simulink model "MotorControlLibNEW"  (R2020b)
settings: Solver=FixedStepDiscrete  StartTime=0.0  StopTime=100  FixedStep=Ts  RelTol=1e-3
values from neighbouring files (symbols this model uses):
  Jm = 0.0000008    (= 8e-07)    [MotorControlLibData.m]    (also in local_pmsm_torque_control_data.m)
  Ld = 1.93E-5    [MotorControl.sldd]    (also in MotorControlLibData.m = 1.93e-05; local_pmsm_torque_control_data.m = 1.93e-05)
  p = 4.0    [MotorControl.sldd]    (also in MotorControlLibData.m = 4; local_pmsm_torque_control_data.m = 4)
  psim = 0.00375    [MotorControl.sldd]    (also in MotorControlLibData.m = 0.00375)
  Rs = 0.022    [MotorControl.sldd]    (also in MotorControlLibData.m = 0.022; local_pmsm_torque_control_data.m = 0.022)
  Ts = 5.0E-5    [MotorControl.sldd]    (also in MotorControlLibData.m = 0.00025; local_pmsm_torque_control_data.m = 5e-06)
  Vnom = 12.0    [MotorControl.sldd]    (also in MotorControlLibData.m = 12; local_pmsm_torque_control_data.m = 12)
undefined symbols (not defined in the file or in its folder): DiscIntNeverNeededParam, Down, Up
libraries: mcbcontrolslib x6, pid_lib x4, eePwmGenerator x3, simulink x2, autolibpmsmexterior x1, eeDqVoltageLimiter x1
settings Model: DataDictionary=MotorControl.sldd  NumberOfSteps=36  Creator=unix  LastModifiedBy=unix
settings SolverCC: AutoInsertRateTranBlk=on

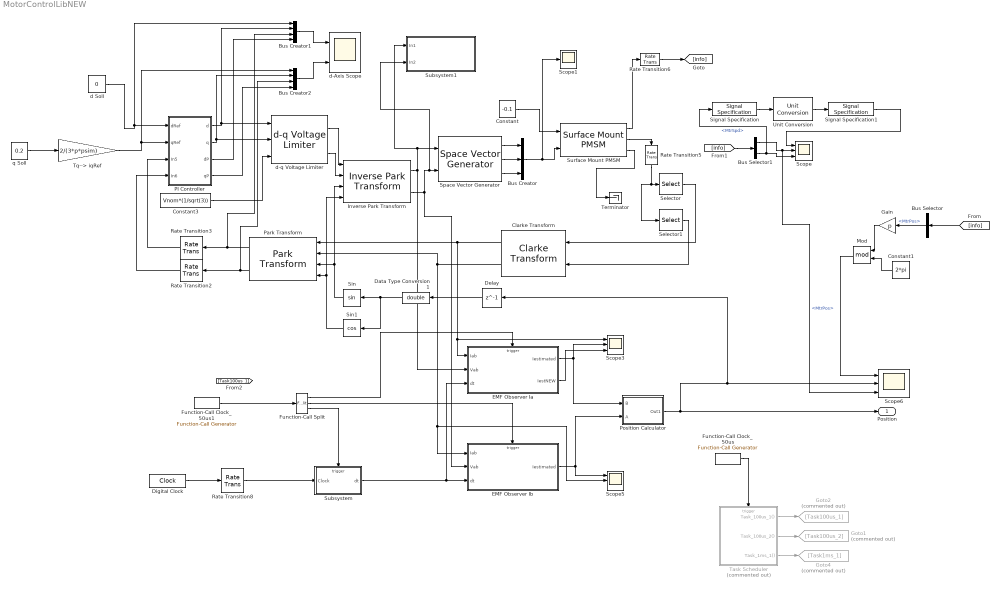
== system MotorControlLibNEW ==
  Bus Creator : BusCreator  Inputs=3
  Bus Creator1 : BusCreator  Inputs=4
  Bus Creator2 : BusCreator  Inputs=4
  Bus Selector : BusSelector  OutputSignals=MtrPos
  Bus Selector1 : BusSelector  OutputSignals=MtrPos,MtrSpd
  Clarke Transform : mcbcontrolslib/Clarke Transform  VariantControl=Variant2
  Constant : Constant  Value=-0.1
  Constant1 : Constant  Value=2*pi
  Constant3 : Constant  Value=Vnom*(1/sqrt(3))
  Data Type Conversion1 : DataTypeConversion  OutDataTypeStr=double
  Delay : Delay  DelayLength=1
  Digital Clock : DigitalClock  SampleTime=Ts
  EMF Observer Ia : Subsystem  mask{Rs=Rs/2, Ld=1/(Ld/2), P=0.255, I=1600}
      mask prompts: Rs "Resistance"; Ld "Inductance"; P "Simulink:masks:ProportionalP_MP"; I "Simulink:masks:IntegralI_MP"
      mask TypeOptions Rs: Resistance/Gain
      mask TypeOptions Ld: Inductance/Gain
      mask TypeOptions P: PID Controller/P
      mask TypeOptions I: PID Controller/I
      mask DialogControl Container6 Prompt: PI Controller
      mask DialogControl P Prompt: Proportional (P):
      mask DialogControl I Prompt: Integral (I):
  EMF Observer Ib : Subsystem  mask{Rs=Rs/2, Ld=1/(Ld/2), P=0.255, I=1600}
      mask prompts: Rs "Resistance"; Ld "Inductance"; P "Simulink:masks:ProportionalP_MP"; I "Simulink:masks:IntegralI_MP"
      mask TypeOptions Rs: Resistance/Gain
      mask TypeOptions Ld: Inductance/Gain
      mask TypeOptions P: PID Controller/P
      mask TypeOptions I: PID Controller/I
      mask DialogControl Container6 Prompt: PI Controller
      mask DialogControl P Prompt: Proportional (P):
      mask DialogControl I Prompt: Integral (I):
  Function-Call Clock_50us : simulink/Ports & Subsystems/Function-Call Generator  sample_time=5e-5  numberOfIterations=1  DisallowWideOutput=off
  Function-Call Clock_50us1 : simulink/Ports & Subsystems/Function-Call Generator  sample_time=Ts  numberOfIterations=1  DisallowWideOutput=off
  Function-Call Split : FunctionCallSplit  IconShape=distinctive  NumOutputPorts=3  OutputPortLayout=default
  Gain : Gain  Gain=p
  Goto1 : Goto  Commented=on  GotoTag=Task100us_2
  Goto2 : Goto  Commented=on  GotoTag=Task100us_1
  Goto4 : Goto  Commented=on  GotoTag=Task1ms_1
  Inverse Park Transform : mcbcontrolslib/Inverse Park Transform  AxisAlignment=D-axis
  Mod : Math  Operator=mod  SaturateOnIntegerOverflow=on
  PI Controller : Subsystem
  Park Transform : mcbcontrolslib/Park Transform  AxisAlignment=D-axis
      settings: SourceProductBaseCode=MT
  Position Calculator : Subsystem
  Rate Transition{2..3,5..6,8} (5 alike) : RateTransition
  Scope{,3,5..6} (4 alike) : Scope  NumInputPorts=3
  Scope1 : Scope
  Selector : Selector  InputPortWidth=3  IndexOptions=Index vector (dialog)  Indices=1  OutputSizes=1
  Selector1 : Selector  InputPortWidth=3  IndexOptions=Index vector (dialog)  Indices=2  OutputSizes=1
  Signal Specification : SignalSpecification  Unit=rad/s
  Signal Specification1 : SignalSpecification  Unit=rpm
  Sin : Trigonometry
  Sin1 : Trigonometry  Operator=cos
  Space Vector Generator : mcbcontrolslib/Space Vector Generator
      settings: SourceProductBaseCode=MT
  Subsystem : Subsystem
  Subsystem1 : Subsystem
  Surface Mount PMSM : autolibpmsmexterior/Surface Mount PMSM  port_config=Torque  sim_type=Discrete  Ts=Ts  P=p  Rs=Rs/2  Ldq_=Ld/2  KConstText=Back-emf constant (Ke):  lambda_pm=0.2205  Ke=cBackEMF_VKPRM  Kt=1.323  mechanical=[Jm, 4.924e-4, 0]  idq0=[0 0]  theta_init=0  omega_init=0  KConst=0.2205  lambda_pm_calc=0.0021651  RefBlkName='autolibpmsmexterior/Surface Mount PMSM'  aMode=5  Ldq="[0.0017      0.0017]"
      settings: SourceProductBaseCode=PW,MT,UV,VE,VP
  Task Scheduler : Stateflow chart  Commented=on  TreatAsAtomicUnit=on
  Terminator : Terminator
  Tq--> iqRef : Gain  Gain=2/(3*p*psim)
  Unit Conversion : UnitConversion
  d Soll : Constant  Value=0
  d-Axis Scope : Scope  NumInputPorts=2
  d-q Voltage Limiter : eeDqVoltageLimiter/d-q Voltage Limiter  AxisPrio=D-axis  Ts=-1
      settings: SourceProductBaseCode=PS
  q Soll : Constant  Value=0.2
  Position : Outport
  wires:
  Constant/1 -> Surface Mount PMSM/1
  Selector1/1 -> Clarke Transform/2
  Selector/1 -> Clarke Transform/1
  Clarke Transform/1 -> Scope3/1, EMF Observer Ia/1(Iab), Park Transform/1
  Clarke Transform/2 -> Park Transform/2, EMF Observer Ib/1(Iab), Scope5/2
  [info] -> Bus Selector/1
  Surface Mount PMSM/1 -> Rate Transition6/1
  Bus Selector/1 -> Gain/1  "<MtrPos>"
  Sin/1 -> Inverse Park Transform/3, Park Transform/3
  Sin1/1 -> Park Transform/4, Inverse Park Transform/4
  Inverse Park Transform/1 -> Subsystem1/1(In1), Space Vector Generator/1, EMF Observer Ia/2(Vab)
  Space Vector Generator/2 -> Bus Creator/2
  Space Vector Generator/3 -> Bus Creator/3
  Bus Selector1/2 -> Signal Specification/1, Scope/3  "<MtrSpd>"
  [info] -> Bus Selector1/1
  Bus Selector1/1 -> Scope6/3, Scope/2  "<MtrPos>"
  Surface Mount PMSM/3 -> Terminator/1
  d-q Voltage Limiter/1 -> Inverse Park Transform/1
  d-q Voltage Limiter/2 -> Inverse Park Transform/2
  Constant3/1 -> d-q Voltage Limiter/3
  Signal Specification1/1 -> Scope/1
  Signal Specification/1 -> Unit Conversion/1
  Unit Conversion/1 -> Signal Specification1/1
  Task Scheduler/1(Task_100us_1()) -> Goto2/1
  Function-Call Clock_50us/1 -> Task Scheduler/Trigger
  Task Scheduler/3(Task_1ms_1()) -> Goto4/1
  Task Scheduler/2(Task_100us_2()) -> Goto1/1
  Inverse Park Transform/2 -> Subsystem1/2(In2), Space Vector Generator/2, EMF Observer Ib/2(Vab)
  Function-Call Split/1 -> EMF Observer Ia/Trigger
  Function-Call Split/2 -> EMF Observer Ib/Trigger
  EMF Observer Ia/1(Iestimated) -> Position Calculator/1(B), Scope3/2
  EMF Observer Ib/1(Iestimated) -> Scope5/1, Position Calculator/2(A)
  Surface Mount PMSM/2 -> Rate Transition5/1
  Data Type Conversion1/1 -> Sin/1, Sin1/1
  Delay/1 -> Data Type Conversion1/1
  Digital Clock/1 -> Rate Transition8/1
  Position Calculator/1(Out1) -> Position/1, Delay/1, Scope6/2
  Subsystem/1(dt) -> EMF Observer Ib/3(dt), EMF Observer Ia/3(dt)
  d Soll/1 -> Bus Creator1/1, PI Controller/1(dRef)
  Tq--> iqRef/1 -> Bus Creator2/1, PI Controller/2(qRef)
  Park Transform/1 -> Bus Creator1/3, Rate Transition3/1
  Park Transform/2 -> Rate Transition2/1, Bus Creator2/3
  PI Controller/1(d) -> d-q Voltage Limiter/1, Bus Creator1/2
  PI Controller/2(q) -> d-q Voltage Limiter/2, Bus Creator2/2
  Rate Transition2/1 -> PI Controller/4(In6)
  Rate Transition3/1 -> PI Controller/3(In5)
  Rate Transition5/1 -> Selector1/1, Selector/1
  Rate Transition6/1 -> [info]
  Rate Transition8/1 -> Subsystem/1(Clock)
  Function-Call Split/3 -> Subsystem/Trigger
  Bus Creator1/1 -> d-Axis Scope/1
  Bus Creator2/1 -> d-Axis Scope/2
  Constant1/1 -> Mod/2
  Gain/1 -> Mod/1
  Mod/1 -> Scope6/1
  PI Controller/3(dP) -> Bus Creator1/4
  PI Controller/4(qP) -> Bus Creator2/4
  q Soll/1 -> Tq--> iqRef/1
  EMF Observer Ia/2(IestNEW) -> Scope3/3
  Function-Call Clock_50us1/1 -> Function-Call Split/1
  Bus Creator/1 -> Scope1/1, Surface Mount PMSM/2
  Space Vector Generator/1 -> Bus Creator/1

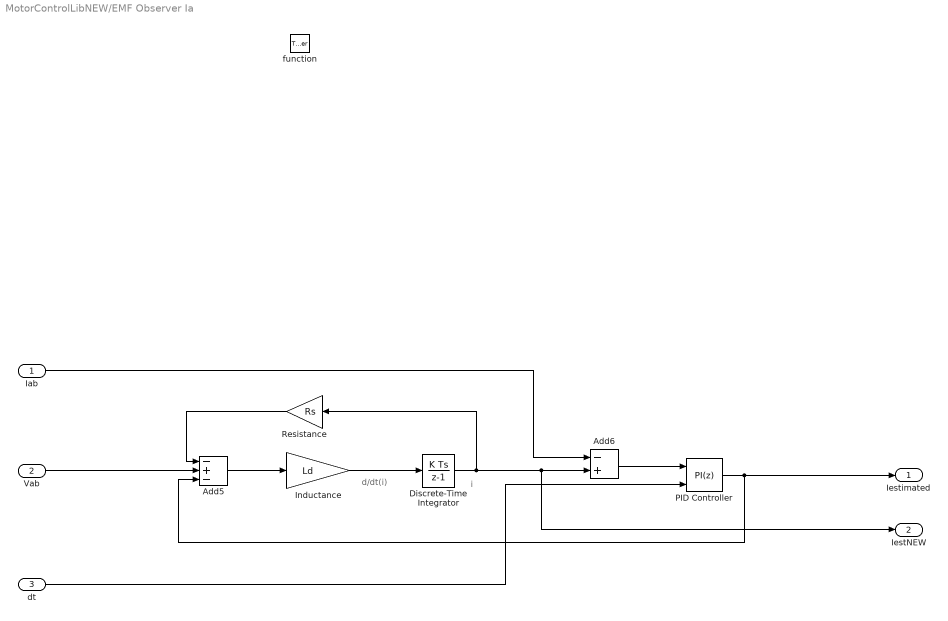
== system MotorControlLibNEW/EMF Observer Ia ==
  note: d/dt(i)
  note: i
  Iab : Inport
  Vab : Inport  Port=2
  dt : Inport  Port=3
  function : TriggerPort  TriggerType=function-call  VariantControl=Variant
  Add5 : Sum  Inputs=-+-
  Add6 : Sum  Inputs=-+
  Discrete-Time Integrator : DiscreteIntegrator  gainval=1  SampleTime=-1  OutDataTypeStr=fixdt(1,32,2^-12,0)  UpperSaturationLimit=18  LowerSaturationLimit=-18  ICPrevOutput=DiscIntNeverNeededParam  ICPrevScaledInput=DiscIntNeverNeededParam
  Inductance : Gain  Gain=Ld
  PID Controller : pid_lib/PID Controller  Controller=PI  Form=Parallel  TimeDomain=Discrete-time  UseExternalTs=on  SampleTime=-1  IntegratorMethod=Forward Euler  FilterMethod=Forward Euler  ControllerParametersSource=internal  P=P  I=I  D=0  UseFilter=on  N=100  TunerSelectOption=Transfer Function Based (PID Tuner App)  InitialConditionSource=internal  InitialConditionForIntegrator=0  InitialConditionForFilter=0  DifferentiatorICPrevScaledInput=0  ExternalReset=none  TrackingMode=off  Kt=1  LimitOutput=off  SatLimitsSource=internal  UpperSaturationLimit=inf  LowerSaturationLimit=-inf  LinearizeAsGain=on  AntiWindupMode=none  Kb=1  POutMin=[]  POutMax=[]  IOutMin=[]  IOutMax=[]  DOutMin=[]  DOutMax=[]  NOutMin=[]  NOutMax=[]  SumOutMin=[]  SumOutMax=[]  SaturationOutMin=[]  SaturationOutMax=[]  PParamMin=[]  PParamMax=[]  IParamMin=[]  IParamMax=[]  DParamMin=[]  DParamMax=[]  NParamMin=[]  NParamMax=[]  KbParamMin=[]  KbParamMax=[]  KtParamMin=[]  KtParamMax=[]  KbOutMin=[]  KbOutMax=[]  KtOutMin=[]  KtOutMax=[]  IntegratorOutMin=[]  IntegratorOutMax=[]  FilterOutMin=[]  FilterOutMax=[]  SumI1OutMin=[]  SumI1OutMax=[]  SumI2OutMin=[]  SumI2OutMax=[]  SumI3OutMin=[]  SumI3OutMax=[]  SumI4OutMin=[]  SumI4OutMax=[]  SumDOutMin=[]  SumDOutMax=[]  DifferentiatorOutMin=[]  DifferentiatorOutMax=[]  FilterDiffOutCoefMin=[]  FilterDiffOutCoefMax=[]  ReciprocalOutMin=[]  ReciprocalOutMax=[]  SumDenOutMin=[]  SumDenOutMax=[]  SumNumOutMin=[]  SumNumOutMax=[]  DivideOutMin=[]  DivideOutMax=[]  UdiffTsProdOutMin=[]  UdiffTsProdOutMax=[]  NTsProdOutMin=[]  NTsProdOutMax=[]  UintegralTsProdOutMin=[]  UintegralTsProdOutMax=[]  UngainTsProdOutMin=[]  UngainTsProdOutMax=[]  IntegratorContinuousStateAttributes=''  IntegratorStateMustResolveToSignalObject=off  IntegratorRTWStateStorageClass=Auto  FilterContinuousStateAttributes=''  FilterStateMustResolveToSignalObject=off  FilterRTWStateStorageClass=Auto  ParallelPVariant=InternalParameters  IdealPVariant=Disabled  IVariant=InternalParameters  DVariant=Disabled  IntegratorVariant=Discrete  SatVariant=Disabled  AWVariant=Passthrough  PCopyVariant=Disabled  TRVariant=Disabled  FdbkBlocksVariant=Forward  IdealPFdbkVariant=Disabled  SatFdbkVariant=Disabled  DerivativeFilterVariant=Disabled  NVariant=Disabled  NCopyVariant=Disabled_SignalSpec  FilterICVariant=Disabled  IntegratorICVariant=InternalICs  ExternalResetVariant=Disabled  TRSumVariant=Passthrough  SumFdbkVariant=Disabled  SumVariant=Sum_PI  TsampFilterVariant=InternalTs  TsampNgainVariant=Passthrough  TsampIntegralVariant=ExternalTs  ExternalSaturationOutDataTypeStr=Inherit: Same as second input
  Resistance : Gain  Gain=Rs
  Iestimated : Outport
  IestNEW : Outport  Port=2
  wires:
  Iab/1 -> Add6/1
  Resistance/1 -> Add5/1
  Add5/1 -> Inductance/1
  Vab/1 -> Add5/2
  Inductance/1 -> Discrete-Time Integrator/1
  Discrete-Time Integrator/1 -> IestNEW/1, Add6/2, Resistance/1
  Add6/1 -> PID Controller/1
  PID Controller/1 -> Add5/3, Iestimated/1
  dt/1 -> PID Controller/2

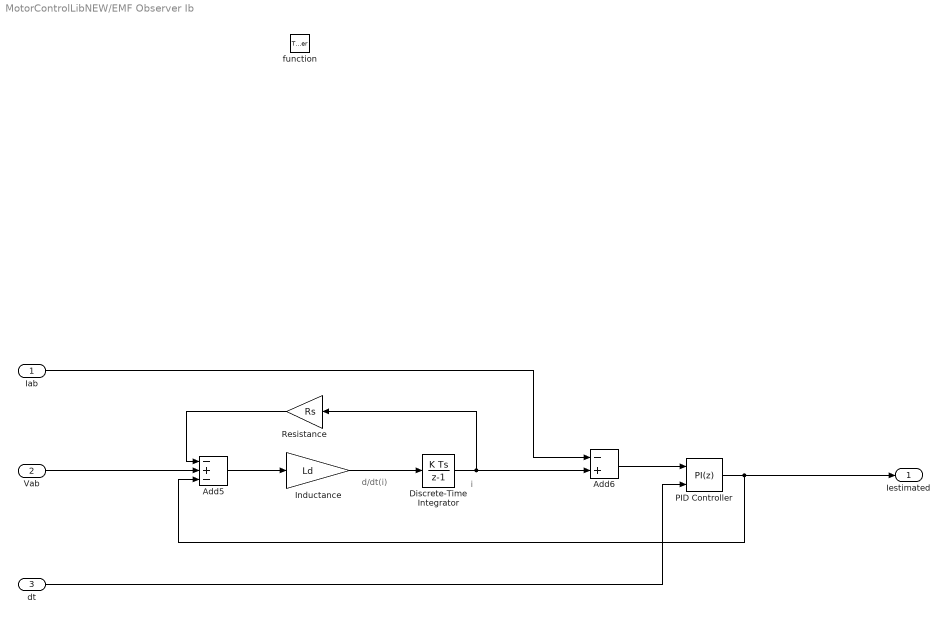
== system MotorControlLibNEW/EMF Observer Ib ==
  note: i
  note: d/dt(i)
  Iab : Inport
  Vab : Inport  Port=2
  dt : Inport  Port=3
  function : TriggerPort  TriggerType=function-call  VariantControl=Variant
  Add5 : Sum  Inputs=-+-
  Add6 : Sum  Inputs=-+
  Discrete-Time Integrator : DiscreteIntegrator  gainval=1  SampleTime=-1  OutDataTypeStr=fixdt(1,32,2^-12,0)  UpperSaturationLimit=18  LowerSaturationLimit=-18  ICPrevOutput=DiscIntNeverNeededParam  ICPrevScaledInput=DiscIntNeverNeededParam
  Inductance : Gain  Gain=Ld
  PID Controller : pid_lib/PID Controller  Controller=PI  Form=Parallel  TimeDomain=Discrete-time  UseExternalTs=on  SampleTime=-1  IntegratorMethod=Forward Euler  FilterMethod=Forward Euler  ControllerParametersSource=internal  P=P  I=I  D=0  UseFilter=on  N=100  TunerSelectOption=Transfer Function Based (PID Tuner App)  InitialConditionSource=internal  InitialConditionForIntegrator=0  InitialConditionForFilter=0  DifferentiatorICPrevScaledInput=0  ExternalReset=none  TrackingMode=off  Kt=1  LimitOutput=off  SatLimitsSource=internal  UpperSaturationLimit=inf  LowerSaturationLimit=-inf  LinearizeAsGain=on  AntiWindupMode=none  Kb=1  POutMin=[]  POutMax=[]  IOutMin=[]  IOutMax=[]  DOutMin=[]  DOutMax=[]  NOutMin=[]  NOutMax=[]  SumOutMin=[]  SumOutMax=[]  SaturationOutMin=[]  SaturationOutMax=[]  PParamMin=[]  PParamMax=[]  IParamMin=[]  IParamMax=[]  DParamMin=[]  DParamMax=[]  NParamMin=[]  NParamMax=[]  KbParamMin=[]  KbParamMax=[]  KtParamMin=[]  KtParamMax=[]  KbOutMin=[]  KbOutMax=[]  KtOutMin=[]  KtOutMax=[]  IntegratorOutMin=[]  IntegratorOutMax=[]  FilterOutMin=[]  FilterOutMax=[]  SumI1OutMin=[]  SumI1OutMax=[]  SumI2OutMin=[]  SumI2OutMax=[]  SumI3OutMin=[]  SumI3OutMax=[]  SumI4OutMin=[]  SumI4OutMax=[]  SumDOutMin=[]  SumDOutMax=[]  DifferentiatorOutMin=[]  DifferentiatorOutMax=[]  FilterDiffOutCoefMin=[]  FilterDiffOutCoefMax=[]  ReciprocalOutMin=[]  ReciprocalOutMax=[]  SumDenOutMin=[]  SumDenOutMax=[]  SumNumOutMin=[]  SumNumOutMax=[]  DivideOutMin=[]  DivideOutMax=[]  UdiffTsProdOutMin=[]  UdiffTsProdOutMax=[]  NTsProdOutMin=[]  NTsProdOutMax=[]  UintegralTsProdOutMin=[]  UintegralTsProdOutMax=[]  UngainTsProdOutMin=[]  UngainTsProdOutMax=[]  IntegratorContinuousStateAttributes=''  IntegratorStateMustResolveToSignalObject=off  IntegratorRTWStateStorageClass=Auto  FilterContinuousStateAttributes=''  FilterStateMustResolveToSignalObject=off  FilterRTWStateStorageClass=Auto  ParallelPVariant=InternalParameters  IdealPVariant=Disabled  IVariant=InternalParameters  DVariant=Disabled  IntegratorVariant=Discrete  SatVariant=Disabled  AWVariant=Passthrough  PCopyVariant=Disabled  TRVariant=Disabled  FdbkBlocksVariant=Forward  IdealPFdbkVariant=Disabled  SatFdbkVariant=Disabled  DerivativeFilterVariant=Disabled  NVariant=Disabled  NCopyVariant=Disabled_SignalSpec  FilterICVariant=Disabled  IntegratorICVariant=InternalICs  ExternalResetVariant=Disabled  TRSumVariant=Passthrough  SumFdbkVariant=Disabled  SumVariant=Sum_PI  TsampFilterVariant=InternalTs  TsampNgainVariant=Passthrough  TsampIntegralVariant=ExternalTs  ExternalSaturationOutDataTypeStr=Inherit: Same as second input
  Resistance : Gain  Gain=Rs
  Iestimated : Outport
  wires:
  dt/1 -> PID Controller/2
  PID Controller/1 -> Iestimated/1, Add5/3
  Add6/1 -> PID Controller/1
  Discrete-Time Integrator/1 -> Resistance/1, Add6/2
  Inductance/1 -> Discrete-Time Integrator/1
  Vab/1 -> Add5/2
  Add5/1 -> Inductance/1
  Resistance/1 -> Add5/1
  Iab/1 -> Add6/1

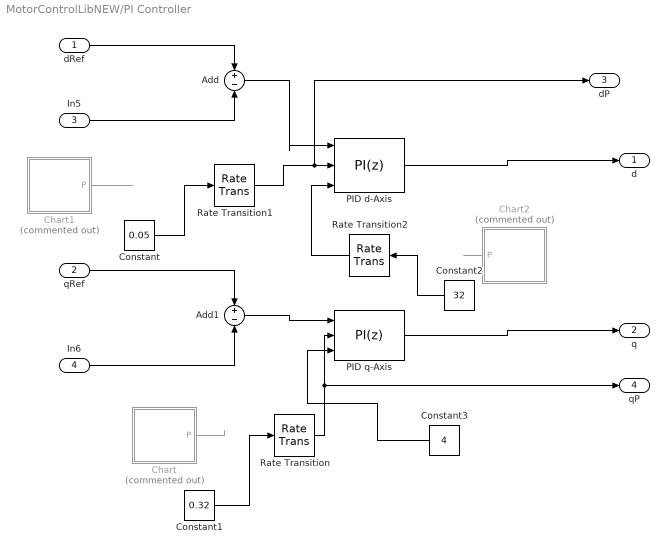
== system MotorControlLibNEW/PI Controller ==
  dRef : Inport
  qRef : Inport  Port=2
  In5 : Inport  Port=3
  In6 : Inport  Port=4
  Add : Sum  Inputs=+|-
  Add1 : Sum  Inputs=+|-
  Chart : Stateflow chart  Commented=on  TreatAsAtomicUnit=on  SystemSampleTime=1000*Ts
  Chart1 : Stateflow chart  Commented=on  TreatAsAtomicUnit=on  SystemSampleTime=1000*Ts
  Chart2 : Stateflow chart  Commented=on  TreatAsAtomicUnit=on  SystemSampleTime=100000*Ts
  Constant : Constant  Value=0.05
  Constant1 : Constant  Value=0.32
  Constant2 : Constant  Value=32
  Constant3 : Constant  Value=4
  PID d-Axis : pid_lib/PID Controller  Controller=PI  Form=Parallel  TimeDomain=Discrete-time  UseExternalTs=off  SampleTime=-1  IntegratorMethod=Forward Euler  FilterMethod=Forward Euler  ControllerParametersSource=external  P=0.1  I=100  D=0  UseFilter=on  N=100  TunerSelectOption=Transfer Function Based (PID Tuner App)  InitialConditionSource=internal  InitialConditionForIntegrator=0  InitialConditionForFilter=0  DifferentiatorICPrevScaledInput=0  ExternalReset=none  TrackingMode=off  Kt=1  LimitOutput=off  SatLimitsSource=internal  UpperSaturationLimit=10  LowerSaturationLimit=-10  LinearizeAsGain=on  AntiWindupMode=none  Kb=1  POutMin=[]  POutMax=[]  IOutMin=[]  IOutMax=[]  DOutMin=[]  DOutMax=[]  NOutMin=[]  NOutMax=[]  SumOutMin=[]  SumOutMax=[]  SaturationOutMin=[]  SaturationOutMax=[]  PParamMin=[]  PParamMax=[]  IParamMin=[]  IParamMax=[]  DParamMin=[]  DParamMax=[]  NParamMin=[]  NParamMax=[]  KbParamMin=[]  KbParamMax=[]  KtParamMin=[]  KtParamMax=[]  KbOutMin=[]  KbOutMax=[]  KtOutMin=[]  KtOutMax=[]  IntegratorOutMin=[]  IntegratorOutMax=[]  FilterOutMin=[]  FilterOutMax=[]  SumI1OutMin=[]  SumI1OutMax=[]  SumI2OutMin=[]  SumI2OutMax=[]  SumI3OutMin=[]  SumI3OutMax=[]  SumI4OutMin=[]  SumI4OutMax=[]  SumDOutMin=[]  SumDOutMax=[]  DifferentiatorOutMin=[]  DifferentiatorOutMax=[]  FilterDiffOutCoefMin=[]  FilterDiffOutCoefMax=[]  ReciprocalOutMin=[]  ReciprocalOutMax=[]  SumDenOutMin=[]  SumDenOutMax=[]  SumNumOutMin=[]  SumNumOutMax=[]  DivideOutMin=[]  DivideOutMax=[]  UdiffTsProdOutMin=[]  UdiffTsProdOutMax=[]  NTsProdOutMin=[]  NTsProdOutMax=[]  UintegralTsProdOutMin=[]  UintegralTsProdOutMax=[]  UngainTsProdOutMin=[]  UngainTsProdOutMax=[]  IntegratorContinuousStateAttributes=''  IntegratorStateMustResolveToSignalObject=off  IntegratorRTWStateStorageClass=Auto  FilterContinuousStateAttributes=''  FilterStateMustResolveToSignalObject=off  FilterRTWStateStorageClass=Auto  ParallelPVariant=ExternalParameters  IdealPVariant=Disabled  IVariant=ExternalParameters  DVariant=Disabled  IntegratorVariant=Discrete  SatVariant=Disabled  AWVariant=Passthrough  PCopyVariant=Disabled  TRVariant=Disabled  FdbkBlocksVariant=Forward  IdealPFdbkVariant=Disabled  SatFdbkVariant=Disabled  DerivativeFilterVariant=Disabled  NVariant=Disabled  NCopyVariant=Disabled_SignalSpec  FilterICVariant=Disabled  IntegratorICVariant=InternalICs  ExternalResetVariant=Disabled  TRSumVariant=Passthrough  SumFdbkVariant=Disabled  SumVariant=Sum_PI  TsampFilterVariant=InternalTs  TsampNgainVariant=Passthrough  TsampIntegralVariant=Passthrough  ExternalSaturationOutDataTypeStr=Inherit: Same as second input
  PID q-Axis : pid_lib/PID Controller  Controller=PI  Form=Parallel  TimeDomain=Discrete-time  UseExternalTs=off  SampleTime=-1  IntegratorMethod=Forward Euler  FilterMethod=Forward Euler  ControllerParametersSource=external  P=0  I=0  D=0  UseFilter=on  N=100  TunerSelectOption=Transfer Function Based (PID Tuner App)  InitialConditionSource=internal  InitialConditionForIntegrator=0  InitialConditionForFilter=0  DifferentiatorICPrevScaledInput=0  ExternalReset=none  TrackingMode=off  Kt=1  LimitOutput=off  SatLimitsSource=internal  UpperSaturationLimit=inf  LowerSaturationLimit=-inf  LinearizeAsGain=on  AntiWindupMode=none  Kb=1  POutMin=[]  POutMax=[]  IOutMin=[]  IOutMax=[]  DOutMin=[]  DOutMax=[]  NOutMin=[]  NOutMax=[]  SumOutMin=[]  SumOutMax=[]  SaturationOutMin=[]  SaturationOutMax=[]  PParamMin=[]  PParamMax=[]  IParamMin=[]  IParamMax=[]  DParamMin=[]  DParamMax=[]  NParamMin=[]  NParamMax=[]  KbParamMin=[]  KbParamMax=[]  KtParamMin=[]  KtParamMax=[]  KbOutMin=[]  KbOutMax=[]  KtOutMin=[]  KtOutMax=[]  IntegratorOutMin=[]  IntegratorOutMax=[]  FilterOutMin=[]  FilterOutMax=[]  SumI1OutMin=[]  SumI1OutMax=[]  SumI2OutMin=[]  SumI2OutMax=[]  SumI3OutMin=[]  SumI3OutMax=[]  SumI4OutMin=[]  SumI4OutMax=[]  SumDOutMin=[]  SumDOutMax=[]  DifferentiatorOutMin=[]  DifferentiatorOutMax=[]  FilterDiffOutCoefMin=[]  FilterDiffOutCoefMax=[]  ReciprocalOutMin=[]  ReciprocalOutMax=[]  SumDenOutMin=[]  SumDenOutMax=[]  SumNumOutMin=[]  SumNumOutMax=[]  DivideOutMin=[]  DivideOutMax=[]  UdiffTsProdOutMin=[]  UdiffTsProdOutMax=[]  NTsProdOutMin=[]  NTsProdOutMax=[]  UintegralTsProdOutMin=[]  UintegralTsProdOutMax=[]  UngainTsProdOutMin=[]  UngainTsProdOutMax=[]  IntegratorContinuousStateAttributes=''  IntegratorStateMustResolveToSignalObject=off  IntegratorRTWStateStorageClass=Auto  FilterContinuousStateAttributes=''  FilterStateMustResolveToSignalObject=off  FilterRTWStateStorageClass=Auto  ParallelPVariant=ExternalParameters  IdealPVariant=Disabled  IVariant=ExternalParameters  DVariant=Disabled  IntegratorVariant=Discrete  SatVariant=Disabled  AWVariant=Passthrough  PCopyVariant=Disabled  TRVariant=Disabled  FdbkBlocksVariant=Forward  IdealPFdbkVariant=Disabled  SatFdbkVariant=Disabled  DerivativeFilterVariant=Disabled  NVariant=Disabled  NCopyVariant=Disabled_SignalSpec  FilterICVariant=Disabled  IntegratorICVariant=InternalICs  ExternalResetVariant=Disabled  TRSumVariant=Passthrough  SumFdbkVariant=Disabled  SumVariant=Sum_PI  TsampFilterVariant=InternalTs  TsampNgainVariant=Passthrough  TsampIntegralVariant=Passthrough  ExternalSaturationOutDataTypeStr=Inherit: Same as second input
  Rate Transition : RateTransition
  Rate Transition1 : RateTransition
  Rate Transition2 : RateTransition
  d : Outport
  q : Outport  Port=2
  dP : Outport  Port=3
  qP : Outport  Port=4
  wires:
  dRef/1 -> Add/1
  qRef/1 -> Add1/1
  In6/1 -> Add1/2
  Add/1 -> PID d-Axis/1
  PID q-Axis/1 -> q/1
  PID d-Axis/1 -> d/1
  In5/1 -> Add/2
  Add1/1 -> PID q-Axis/1
  Chart/1(P) -> ?
  Rate Transition/1 -> qP/1, PID q-Axis/2
  Chart1/1(P) -> ?
  Rate Transition1/1 -> dP/1, PID d-Axis/2
  Chart2/1(P) -> ?
  Rate Transition2/1 -> PID d-Axis/3
  Constant1/1 -> Rate Transition/1
  Constant/1 -> Rate Transition1/1
  Constant2/1 -> Rate Transition2/1
  Constant3/1 -> PID q-Axis/3

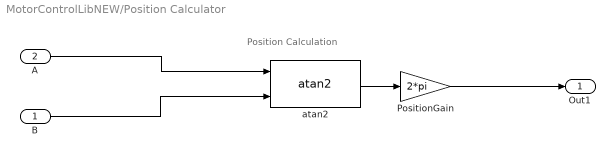
== system MotorControlLibNEW/Position Calculator ==
  note: Position Calculation
  B : Inport
  A : Inport  Port=2
  PositionGain : Gain  Gain=2*pi  OutDataTypeStr=single  RndMeth=Simplest
  atan2 : mcbcontrolslib/atan2  outputUnit=PerUnit
      settings: SourceProductBaseCode=MT
  Out1 : Outport
  wires:
  A/1 -> atan2/1
  PositionGain/1 -> Out1/1
  atan2/1 -> PositionGain/1
  B/1 -> atan2/2

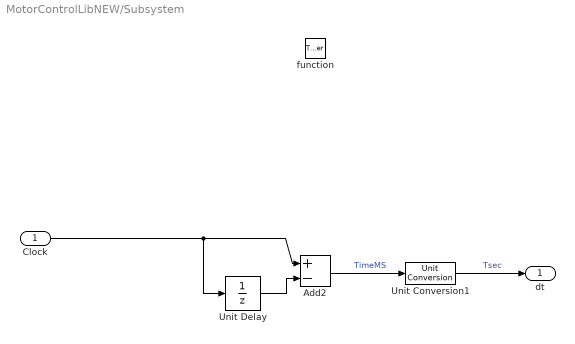
== system MotorControlLibNEW/Subsystem ==
  Clock : Inport
  function : TriggerPort  TriggerType=function-call  VariantControl=Variant
  Add2 : Sum  Inputs=+-
  Unit Conversion1 : UnitConversion  OutputType=Inherit: Inherit via back propagation
  Unit Delay : UnitDelay  SampleTime=-1  HasFrameUpgradeWarning=on
  dt : Outport
  wires:
  Add2/1 -> Unit Conversion1/1  "TimeMS"
  Unit Delay/1 -> Add2/2
  Clock/1 -> Unit Delay/1, Add2/1
  Unit Conversion1/1 -> dt/1  "Tsec"

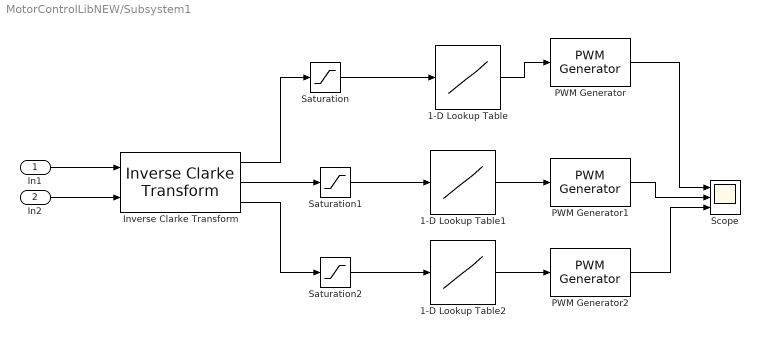
== system MotorControlLibNEW/Subsystem1 ==
  In1 : Inport
  In2 : Inport  Port=2
  1-D Lookup Table : Lookup_n-D  NumberOfTableDimensions=1  BreakpointsForDimension1=[-(sqrt(3)/2)*12 0 (sqrt(3)/2)*12]  Table=[0 0.5 1]  InternalRulePriority=Speed  RndMeth=Simplest  InputSameDT=on
  1-D Lookup Table1 : Lookup_n-D  NumberOfTableDimensions=1  BreakpointsForDimension1=[-(sqrt(3)/2)*12 0 (sqrt(3)/2)*12]  Table=[0 0.5 1]  InternalRulePriority=Speed  RndMeth=Simplest  InputSameDT=on
  1-D Lookup Table2 : Lookup_n-D  NumberOfTableDimensions=1  BreakpointsForDimension1=[-(sqrt(3)/2)*12 0 (sqrt(3)/2)*12]  Table=[0 0.5 1]  InternalRulePriority=Speed  RndMeth=Simplest  InputSameDT=on
  Inverse Clarke Transform : mcbcontrolslib/Inverse Clarke Transform
      settings: SourceProductBaseCode=MT
  PWM Generator : eePwmGenerator/PWM Generator  CarrCount=Up-Down  Tper=1e-4  Ts=5e-6
  PWM Generator1 : eePwmGenerator/PWM Generator  CarrCount=Up-Down  Tper=1e-4  Ts=5e-6
  PWM Generator2 : eePwmGenerator/PWM Generator  CarrCount=Up-Down  Tper=1e-4  Ts=5e-6
  Saturation : Saturate  UpperLimit=(sqrt(3)/2)*12  LowerLimit=-(sqrt(3)/2)*12
  Saturation1 : Saturate  UpperLimit=(sqrt(3)/2)*12  LowerLimit=-(sqrt(3)/2)*12
  Saturation2 : Saturate  UpperLimit=(sqrt(3)/2)*12  LowerLimit=-(sqrt(3)/2)*12
  Scope : Scope  NumInputPorts=3
  wires:
  In2/1 -> Inverse Clarke Transform/2
  In1/1 -> Inverse Clarke Transform/1
  Inverse Clarke Transform/1 -> Saturation/1
  Saturation/1 -> 1-D Lookup Table/1
  1-D Lookup Table/1 -> PWM Generator/1
  Saturation1/1 -> 1-D Lookup Table1/1
  Inverse Clarke Transform/2 -> Saturation1/1
  Saturation2/1 -> 1-D Lookup Table2/1
  Inverse Clarke Transform/3 -> Saturation2/1
  PWM Generator/1 -> Scope/1
  1-D Lookup Table2/1 -> PWM Generator2/1
  1-D Lookup Table1/1 -> PWM Generator1/1
  PWM Generator1/1 -> Scope/2
  PWM Generator2/1 -> Scope/3

== stateflow chart MotorControlLibNEW/Task Scheduler ==
  (default) -> (junction 23) : CLK_50us
  (junction 23) -> (junction 17)
  (junction 17) -> (junction 22) [order 2]
  (junction 17) -> (junction 22) [order 1] : [cnt%%2==0]{Task_100us_1;}
  (junction 22) -> (junction 18) [order 2]
  (junction 22) -> (junction 18) [order 1] : [cnt%%2==0]{Task_100us_2;}
  (junction 18) -> (junction 21) [order 1] : [cnt%%20==0]{Task_1ms_1;}
  (junction 18) -> (junction 21) [order 2]
  (junction 21) -> (junction 34) [order 2]
  (junction 21) -> (junction 16) [order 1] : [1]{cnt++;}
  data: cnt local int32
  events: Task_100us_1 output FUNCTION_CALL_EVENT; Task_100us_2 output FUNCTION_CALL_EVENT; Task_1ms_1 output FUNCTION_CALL_EVENT; CLK_50us input FUNCTION_CALL_EVENT

== stateflow chart MotorControlLibNEW/PI Controller/Chart1 ==
  (default) -> (junction 6) : /* P Value ++ */
  (junction 6) -> (junction 19) [order 1] : [P==0]{P=0.00;}
  (junction 6) -> (junction 17) [order 2]
  (junction 19) -> (junction 17)
  (junction 17) -> (junction 24) [order 2]
  (junction 17) -> (junction 8) [order 1] : {P+=0.01;}
  (junction 8) -> (junction 11) [order 2] : [P<=0]
  (junction 11) -> (junction 13)
  (junction 8) -> (junction 9) [order 1] : [P>0]{P=0.15;}
  (junction 9) -> (junction 13)
  data: P output double

== stateflow chart MotorControlLibNEW/PI Controller/Chart ==
  (default) -> (junction 6) : /* P Value ++ */
  (junction 6) -> (junction 8) : {P+=0.001;}
  (junction 8) -> (junction 11) [order 2] : [P<=0]
  (junction 11) -> (junction 13)
  (junction 8) -> (junction 9) [order 1] : [P>0]{P=0.02;}
  (junction 9) -> (junction 13)
  data: P output double

== stateflow chart MotorControlLibNEW/PI Controller/Chart2 ==
  (default) -> (junction 6) : /* P Value ++ */
  (junction 6) -> (junction 8) : {P+=1;}
  (junction 8) -> (junction 11) [order 2] : [P<=0]
  (junction 11) -> (junction 13)
  (junction 8) -> (junction 9) [order 1] : [P>0]{P=4;}
  (junction 9) -> (junction 13)
  data: P output double
